simulink model "StewartPlatform"  (R2015a)
settings: Solver=ode45  StartTime=0.0  StopTime=10.0  RelTol=1e-3
libraries: aerolibutil x3, vrlib x1
settings Model: Creator=admin  LastModifiedBy=admin

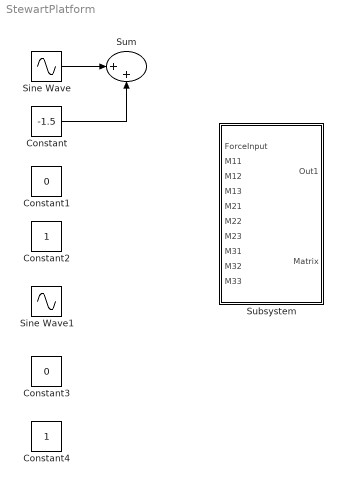
== system StewartPlatform ==
  Constant : Constant  Value=-1.5
  Constant1 : Constant  Value=0
  Constant2 : Constant
  Constant3 : Constant  Value=0
  Constant4 : Constant
  Sine Wave : Sin  Amplitude=0.1  Frequency=3.14  SampleTime=0
  Sine Wave1 : Sin  Amplitude=0.1  Frequency=3.14  SampleTime=0
  Subsystem : Subsystem
  Sum : Sum  Inputs=|++
  wires:
  Sine Wave/1 -> Sum/1
  Constant/1 -> Sum/2

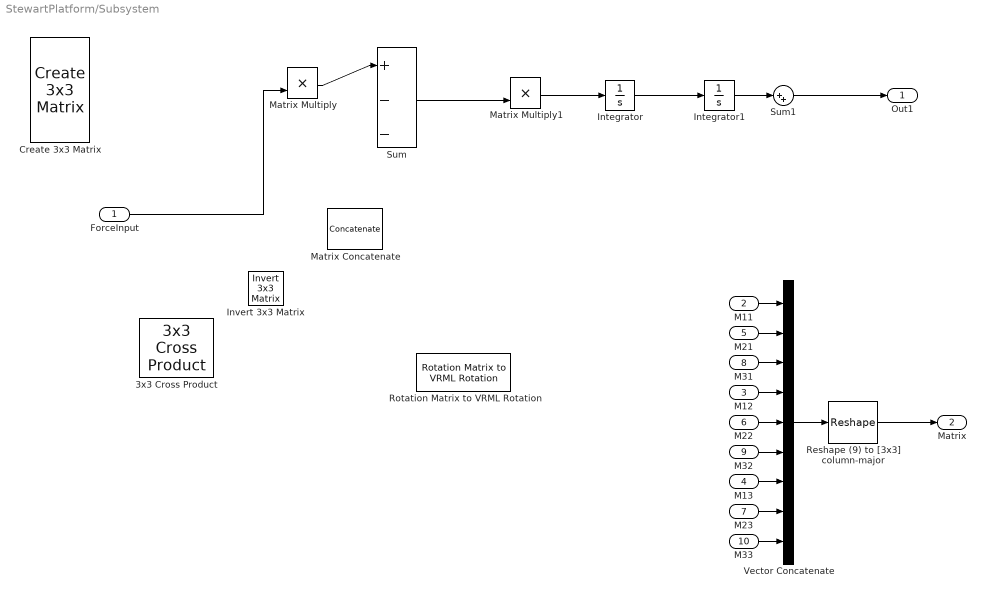
== system StewartPlatform/Subsystem ==
  ForceInput : Inport
  M11 : Inport  Port=2  PortDimensions=1
  M12 : Inport  Port=3  PortDimensions=1
  M13 : Inport  Port=4  PortDimensions=1
  M21 : Inport  Port=5  PortDimensions=1
  M22 : Inport  Port=6  PortDimensions=1
  M23 : Inport  Port=7  PortDimensions=1
  M31 : Inport  Port=8  PortDimensions=1
  M32 : Inport  Port=9  PortDimensions=1
  M33 : Inport  Port=10  PortDimensions=1
  3x3 Cross Product : aerolibutil/3x3 Cross Product
  Create 3x3 Matrix : aerolibutil/Create 3x3 Matrix
  Integrator : Integrator
  Integrator1 : Integrator
  Invert 3x3 Matrix : aerolibutil/Invert  3x3 Matrix
  Matrix Concatenate : Concatenate  Mode=Multidimensional array  ConcatenateDimension=2
  Matrix Multiply : Product
  Matrix Multiply1 : Product
  Reshape (9) to [3x3] column-major : Reshape  OutputDimensionality=Customize  OutputDimensions=[3,3]
  Rotation Matrix to VRML Rotation : vrlib/Utilities/Rotation Matrix to VRML Rotation  maxzero=1e-12
  Sum : Sum  Inputs=|+--
  Sum1 : Sum  Inputs=|++
  Vector Concatenate : Concatenate  NumInputs=9
  Out1 : Outport
  Matrix : Outport  Port=2  PortDimensions=[3 3]
  wires:
  ForceInput/1 -> Matrix Multiply/2
  Matrix Multiply/1 -> Sum/1
  Sum/1 -> Matrix Multiply1/2
  Matrix Multiply1/1 -> Integrator/1
  Integrator/1 -> Integrator1/1
  Integrator1/1 -> Sum1/1
  Sum1/1 -> Out1/1
  M33/1 -> Vector Concatenate/9
  M23/1 -> Vector Concatenate/8
  M13/1 -> Vector Concatenate/7
  M32/1 -> Vector Concatenate/6
  Reshape (9) to [3x3] column-major/1 -> Matrix/1
  M22/1 -> Vector Concatenate/5
  M12/1 -> Vector Concatenate/4
  M31/1 -> Vector Concatenate/3
  M21/1 -> Vector Concatenate/2
  M11/1 -> Vector Concatenate/1
  Vector Concatenate/1 -> Reshape (9) to [3x3] column-major/1
